simulink model "model_2_2018b"  (R2018b)
settings: Solver=VariableStepAuto  StartTime=0.0  StopTime=50  MaxStep=0.01  RelTol=1e-3
undefined symbols (not defined in the file): X, Y, Z
libraries: sm_lib x28, nesl_utility x13, simulink x7
(part 2 of 2)

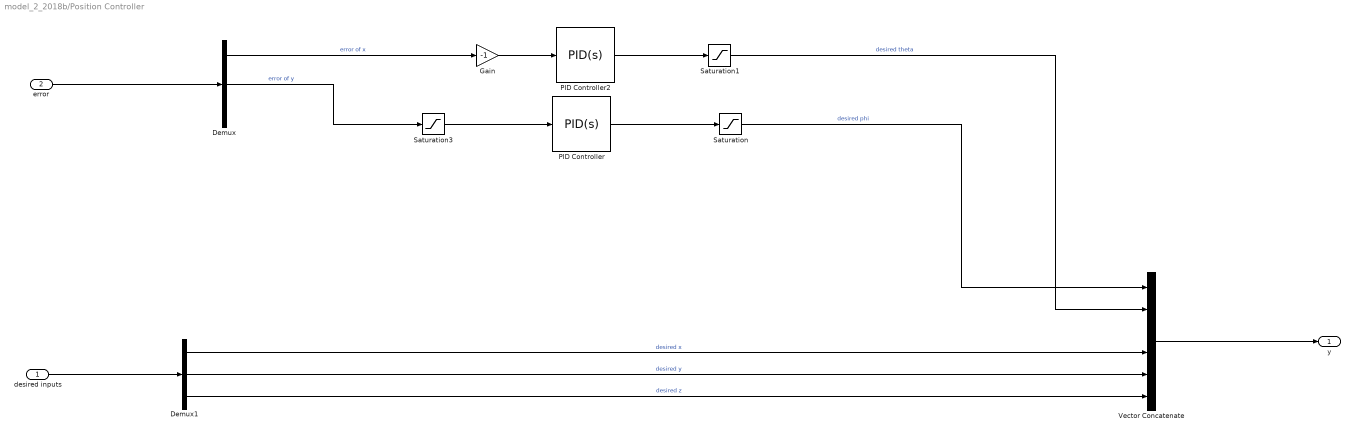
== system model_2_2018b/Position Controller ==
  desired inputs : Inport
  error : Inport  Port=2
  Demux : Demux  Outputs=3
  Demux1 : Demux  Outputs=3
  Gain : Gain  Gain=-1
  PID Controller : simulink/Continuous/PID Controller  Controller=PID  Form=Parallel  TimeDomain=Continuous-time  SampleTime=-1  IntegratorMethod=Forward Euler  ControllerParametersSource=internal  P=0.003  I=0  D=0.007  UseFilter=on  N=100  TunerSelectOption=Transfer Function Based (PID Tuner App)  InitialConditionSource=internal  InitialConditionForIntegrator=0  InitialConditionForFilter=0  DifferentiatorICPrevScaledInput=0  ExternalReset=none  TrackingMode=off  Kt=1  LimitOutput=off  UpperSaturationLimit=inf  LowerSaturationLimit=-inf  LinearizeAsGain=on  AntiWindupMode=none  Kb=1  POutMin=[]  POutMax=[]  IOutMin=[]  IOutMax=[]  DOutMin=[]  DOutMax=[]  NOutMin=[]  NOutMax=[]  SumOutMin=[]  SumOutMax=[]  SaturationOutMin=[]  SaturationOutMax=[]  PParamMin=[]  PParamMax=[]  IParamMin=[]  IParamMax=[]  DParamMin=[]  DParamMax=[]  NParamMin=[]  NParamMax=[]  KbParamMin=[]  KbParamMax=[]  KtParamMin=[]  KtParamMax=[]  KbOutMin=[]  KbOutMax=[]  KtOutMin=[]  KtOutMax=[]  IntegratorOutMin=[]  IntegratorOutMax=[]  FilterOutMin=[]  FilterOutMax=[]  SumI1OutMin=[]  SumI1OutMax=[]  SumI2OutMin=[]  SumI2OutMax=[]  SumI3OutMin=[]  SumI3OutMax=[]  SumI4OutMin=[]  SumI4OutMax=[]  SumDOutMin=[]  SumDOutMax=[]  DifferentiatorOutMin=[]  DifferentiatorOutMax=[]  FilterDiffOutCoefMin=[]  FilterDiffOutCoefMax=[]  ReciprocalOutMin=[]  ReciprocalOutMax=[]  SumDenOutMin=[]  SumDenOutMax=[]  SumNumOutMin=[]  SumNumOutMax=[]  DivideOutMin=[]  DivideOutMax=[]  IntegratorContinuousStateAttributes=''  IntegratorStateMustResolveToSignalObject=off  IntegratorRTWStateStorageClass=Auto  FilterContinuousStateAttributes=''  FilterStateMustResolveToSignalObject=off  FilterRTWStateStorageClass=Auto  ParallelPVariant=InternalParameters  IdealPVariant=Disabled  IVariant=InternalParameters  DVariant=InternalParameters  IntegratorVariant=Continuous  SatVariant=Disabled  AWVariant=Passthrough  PCopyVariant=Disabled  TRVariant=Disabled  FdbkBlocksVariant=Forward  IdealPFdbkVariant=Disabled  SatFdbkVariant=Disabled  DerivativeFilterVariant=ContFilter  NVariant=InternalParameters  NCopyVariant=Disabled  FilterICVariant=InternalICsFilter  IntegratorICVariant=InternalICs  ExternalResetVariant=Disabled  TRSumVariant=Passthrough  SumFdbkVariant=Disabled  SumVariant=Sum_PID
  PID Controller2 : simulink/Continuous/PID Controller  Controller=PID  Form=Parallel  TimeDomain=Continuous-time  SampleTime=-1  IntegratorMethod=Forward Euler  ControllerParametersSource=internal  P=0.0001  I=0  D=0.00001  UseFilter=on  N=100  TunerSelectOption=Transfer Function Based (PID Tuner App)  InitialConditionSource=internal  InitialConditionForIntegrator=0  InitialConditionForFilter=0  DifferentiatorICPrevScaledInput=0  ExternalReset=none  TrackingMode=off  Kt=1  LimitOutput=off  UpperSaturationLimit=inf  LowerSaturationLimit=-inf  LinearizeAsGain=on  AntiWindupMode=none  Kb=1  POutMin=[]  POutMax=[]  IOutMin=[]  IOutMax=[]  DOutMin=[]  DOutMax=[]  NOutMin=[]  NOutMax=[]  SumOutMin=[]  SumOutMax=[]  SaturationOutMin=[]  SaturationOutMax=[]  PParamMin=[]  PParamMax=[]  IParamMin=[]  IParamMax=[]  DParamMin=[]  DParamMax=[]  NParamMin=[]  NParamMax=[]  KbParamMin=[]  KbParamMax=[]  KtParamMin=[]  KtParamMax=[]  KbOutMin=[]  KbOutMax=[]  KtOutMin=[]  KtOutMax=[]  IntegratorOutMin=[]  IntegratorOutMax=[]  FilterOutMin=[]  FilterOutMax=[]  SumI1OutMin=[]  SumI1OutMax=[]  SumI2OutMin=[]  SumI2OutMax=[]  SumI3OutMin=[]  SumI3OutMax=[]  SumI4OutMin=[]  SumI4OutMax=[]  SumDOutMin=[]  SumDOutMax=[]  DifferentiatorOutMin=[]  DifferentiatorOutMax=[]  FilterDiffOutCoefMin=[]  FilterDiffOutCoefMax=[]  ReciprocalOutMin=[]  ReciprocalOutMax=[]  SumDenOutMin=[]  SumDenOutMax=[]  SumNumOutMin=[]  SumNumOutMax=[]  DivideOutMin=[]  DivideOutMax=[]  IntegratorContinuousStateAttributes=''  IntegratorStateMustResolveToSignalObject=off  IntegratorRTWStateStorageClass=Auto  FilterContinuousStateAttributes=''  FilterStateMustResolveToSignalObject=off  FilterRTWStateStorageClass=Auto  ParallelPVariant=InternalParameters  IdealPVariant=Disabled  IVariant=InternalParameters  DVariant=InternalParameters  IntegratorVariant=Continuous  SatVariant=Disabled  AWVariant=Passthrough  PCopyVariant=Disabled  TRVariant=Disabled  FdbkBlocksVariant=Forward  IdealPFdbkVariant=Disabled  SatFdbkVariant=Disabled  DerivativeFilterVariant=ContFilter  NVariant=InternalParameters  NCopyVariant=Disabled  FilterICVariant=InternalICsFilter  IntegratorICVariant=InternalICs  ExternalResetVariant=Disabled  TRSumVariant=Passthrough  SumFdbkVariant=Disabled  SumVariant=Sum_PID
  Saturation : Saturate  UpperLimit=1.57  LowerLimit=-1.57
  Saturation1 : Saturate  UpperLimit=1.57  LowerLimit=-1.57
  Saturation3 : Saturate  UpperLimit=20  LowerLimit=-20
  Vector Concatenate : Concatenate  NumInputs=6
  y : Outport  PortDimensions=6
  wires:
  error/1 -> Demux/1
  Vector Concatenate/1 -> y/1
  Demux/2 -> Saturation3/1  "error of y"
  desired inputs/1 -> Demux1/1
  Demux1/3 -> Vector Concatenate/6  "desired z"
  Demux1/2 -> Vector Concatenate/5  "desired y"
  Demux1/1 -> Vector Concatenate/4  "desired x"
  PID Controller/1 -> Saturation/1
  Saturation/1 -> Vector Concatenate/1  "desired phi"
  PID Controller2/1 -> Saturation1/1
  Saturation1/1 -> Vector Concatenate/2  "desired theta"
  Gain/1 -> PID Controller2/1
  Demux/1 -> Gain/1  "error of x"
  Saturation3/1 -> PID Controller/1

== matlab function model_2_2018b/Mixer ==
  data: Mx input; w1 output; w2 output; My input; Mz input; fx input; w3 output; w4 output; gama1 output; gama2 output; fz input; g1 input; g2 input
function [w1,w2,w3,w4,gama1,gama2] = fcn(Mx,My,Mz,fx,fz,g1,g2)
% both M and f should be in body's coordinate
m = 5;
g = 9.81;
CT = 0.02;
Cm = 0.005;
b = 0.25;
T1=10;  T2=10;  T3=10;  T4=10;
gama1=g1; gama2=g2;
%gama1=0; gama2=0;
i=0;
eps=1e-3;
del=100*eps;
while del>eps 
    c1=cos(gama1); c2=cos(gama2); s1=sin(gama1); s2=sin(gama2);
    AB =[-b*c1-Cm/CT*s1, b*c2+Cm/CT*s2,    b,   -b;
        b*c1,          b*c2,             -b,      -b;
        -b*s1+Cm/CT*c1, b*s2-Cm/CT*c2,     Cm/CT,  -Cm/CT;
         s1,            s2,                0,       0;
         -c1,          -c2,               -1,      -1];
    
    T = abs( AB\[Mx;My;Mz;fx;fz]);%%%%%%%% abs
    T1=T(1);  T2=T(2);  T3=T(3);  T4=T(4);
    
    gama1 = atan2( fx-T2*sin(gama2) , -fz-T3-T4-T2*cos(gama2) );
    gama2 = atan2( fx-T1*sin(gama1) , -fz-T3-T4-T1*cos(gama1) );
     del = abs( fx -T2*sin(gama2)-T1*sin(gama1) )...
         + abs( fz+T2*cos(gama2)+T1*cos(gama1)+T3+T4 );
    i=i+1;
    if i>200
        gama1=g1; gama2=g2;
        break
    end
    %disp(del); disp(i);
end

w1 = sqrt(T1/(0.5*CT));
w2 = sqrt(T2/(0.5*CT));
w3 = sqrt(T3/(0.5*CT));
w4 = sqrt(T4/(0.5*CT));
% w1 = T1;
% w2 = T2;
% w3 = T3;
% w4 = T4;

if abs(gama1)>2 || abs(gama2)>2
    gama1=0; gama2=0;
end
end

== matlab function model_2_2018b/Plant ==
  data: phi_ output; theta_ output; psi_ output; gama_1 output; gama_2 output; phi output; theta output; psi output; X_dd output; w1 input; w2 input; w3 input; w4 input; q0 input; q1 input; q2 input; q3 input; w_d output; w input; q0_d output; q1_d output; q2_d output; q3_d output; gama1 input; gama2 input
function [phi_,theta_,psi_,gama_1,gama_2,phi,theta,psi,X_dd,w_d,q0_d,q1_d,q2_d,q3_d]= fcn( w1, w2, w3, w4, q0, q1,  q2, q3, w, gama1, gama2)
m = 5;
g = 9.81;
CT = 0.02;
Cm = 0.005;
b = 0.25;

T1 = 0.5*CT*w1^2;
T2 = 0.5*CT*w2^2;
T3 = 0.5*CT*w3^2;
T4 = 0.5*CT*w4^2;


R_I_b = [ q0^2+q1^2-q2^2-q3^2 , 2*(q1*q2 + q0*q3), 2*(q1*q3-q0*q2);
       2*(q1*q2-q0*q3), q0^2-q1^2+q2^2-q3^2 , 2*(q2*q3+q0*q1);
       2*(q1*q3+q0*q2) , 2*(q2*q3-q0*q1), q0^2-q1^2-q2^2+q3^2 ];
   
R_b_I = R_I_b';
F = R_b_I * [T1*sin(gama1)+T2*sin(gama2);0;-(T1*cos(gama1)+T2*cos(gama2)+T3+T4)];

X_dd = (F+[0;0;m*g])/m;

I = [ 1     0  0.2;
      0     1   0 ;
     0.2    0  1.5 ];
 
p = w(1); q = w(2); r = w(3);

Sw = [0 -r  q;...
      r  0 -p;...
     -q  p  0];

M = [b*( -T1*cos(gama1)+T2*cos(gama2)+T3-T4 ) + Cm/CT*( -T1*sin(gama1)+T2*sin(gama2) );...
     b*( T1*cos(gama1)+T2*cos(gama2)-T3-T4 );...
     Cm/CT *( T1*cos(gama1)-T2*cos(gama2)+T3-T4 ) + b*T2*sin(gama2) - b*T1*sin(gama1)];
 
w_d = I\(M - Sw*I*w);

G=0.5*[0 -p -q -r;
       p  0  r -q;
       q -r  0  p;
       r  q -p  0];
   
q_d = G*[q0;q1;q2;q3];
q0_d=q_d(1);
q1_d=q_d(2);
q2_d=q_d(3);
q3_d=q_d(4);

phi=atan(2*(q0*q1+q2*q3)/(1-2*(q1^2+q2^2)));
theta=real(asin(complex(2*(q0*q2-q1*q3))));
psi=atan(2*(q0*q3+q1*q2)/(1-2*(q2^2+q3^2)));
gama_1 = gama1;
gama_2 = gama2;

angles = quat2eul([q0,q1,q2,q3],'XYZ');
phi_=angles(1); theta_=angles(2); psi_=angles(3);

end

== matlab function model_2_2018b/Inertia to body transformer ==
  data: input input; y output; q0 input; q1 input; q2 input; q3 input
function y = fcn(input,q0,q1,q2,q3)
xI=input(4); yI=input(5); zI=input(6); 
XI=[xI;yI;zI];
R_I_b = [ q0^2+q1^2-q2^2-q3^2 , 2*(q1*q2 + q0*q3), 2*(q1*q3-q0*q2);
       2*(q1*q2-q0*q3), q0^2-q1^2+q2^2-q3^2 , 2*(q2*q3+q0*q1);
       2*(q1*q3+q0*q2) , 2*(q2*q3-q0*q1), q0^2-q1^2-q2^2+q3^2 ];
Xb = R_I_b*XI;

y = [input(1); input(2); input(3); Xb(1); Xb(2); Xb(3)];
end

== matlab function model_2_2018b/Inertia to body transformer_3 par ==
  data: input input; y output; q0 input; q1 input; q2 input; q3 input
function y = fcn(input,q0,q1,q2,q3)
xI=input(1); yI=input(2); zI=input(3); 
XI=[xI;yI;zI];
R_I_b = [ q0^2+q1^2-q2^2-q3^2 , 2*(q1*q2 + q0*q3), 2*(q1*q3-q0*q2);
       2*(q1*q2-q0*q3), q0^2-q1^2+q2^2-q3^2 , 2*(q2*q3+q0*q1);
       2*(q1*q3+q0*q2) , 2*(q2*q3-q0*q1), q0^2-q1^2-q2^2+q3^2 ];
Xb = R_I_b*XI;

% y1=Xb(1);
% y2=Xb(2);
% y3=Xb(3);
y = [Xb(1); Xb(2); Xb(3) ];

end

== matlab function model_2_2018b/Attitude Controller/MATLAB Function ==
  data: u input; y output
function y = fcn(u)

y = wrapToPi(u);
